simulink model "atlas_joint_impctrl_sqrt_damping_test"  (Simulink 8.5)
settings: Solver=ode4  StartTime=0.0  StopTime=2.0  FixedStep=1e-4  RelTol=1e-3
values from neighbouring files (symbols this model uses):
  B = d - 0.1*ones(NJL,1)    [atlas_joint_impctrl_sqrt_damping_test_settings_default.m]
  D = 0.7*eye(NJL)    [atlas_joint_impctrl_sqrt_damping_test_settings_default.m]
  F_ext_noise = 3    [atlas_joint_impctrl_sqrt_damping_test_settings_default.m]
  F_ext_noise_seed = 0    [atlas_joint_impctrl_sqrt_damping_test_settings_default.m]
  F_ext_noise_switch = 0    [atlas_joint_impctrl_sqrt_damping_test_settings_default.m]
  g_noise = 0.001    [atlas_joint_impctrl_sqrt_damping_test_settings_default.m]
  g_noise_seed = 0    [atlas_joint_impctrl_sqrt_damping_test_settings_default.m]
  g_noise_switch = 0    [atlas_joint_impctrl_sqrt_damping_test_settings_default.m]
  q_noise = 0.01    [atlas_joint_impctrl_sqrt_damping_test_settings_default.m]
  q_noise_seed = 0    [atlas_joint_impctrl_sqrt_damping_test_settings_default.m]
  q_noise_switch = 0    [atlas_joint_impctrl_sqrt_damping_test_settings_default.m]
  qD_noise = 0.01    [atlas_joint_impctrl_sqrt_damping_test_settings_default.m]
  qD_noise_seed = 0    [atlas_joint_impctrl_sqrt_damping_test_settings_default.m]
  qD_noise_switch = 0    [atlas_joint_impctrl_sqrt_damping_test_settings_default.m]
  T = 0.001    [atlas_joint_impctrl_sqrt_damping_test_settings_default.m]
  tau_noise = 0.5    [atlas_joint_impctrl_sqrt_damping_test_settings_default.m]
  tau_noise_seed = 0    [atlas_joint_impctrl_sqrt_damping_test_settings_default.m]
  tau_noise_switch = 0    [atlas_joint_impctrl_sqrt_damping_test_settings_default.m]
undefined symbols (not defined in the file): T1_filter_input, T1_filter_output
libraries: atlas_dynamic_library x5, atlas_impctrl_library x2
settings Model: Creator=knoechelmann  LastModifiedBy=Vorndamme  SimulationMode=rapid-accelerator  CovSFcnEnable=off
settings DataIOCC: LimitDataPoints=off  SaveFormat=StructureWithTime  SignalLoggingSaveFormat=Dataset
settings OptimizationCC: ExpressionDepthLimit=128
settings DebuggingCC: SignalInfNanChecking=warning  SignalRangeChecking=warning  UnderspecifiedInitializationDetection=Simplified  MergeDetectMultiDrivingBlocksExec=error  SolverPrmCheckMsg=warning  MultiTaskRateTransMsg=warning  CheckMatrixSingularityMsg=warning  UnderSpecifiedDataTypeMsg=warning  FcnCallInpInsideContextMsg=EnableAllAsError  StateNameClashWarn=none
settings GRTTargetCC: CombineOutputUpdateFcns=on  GRTInterface=off

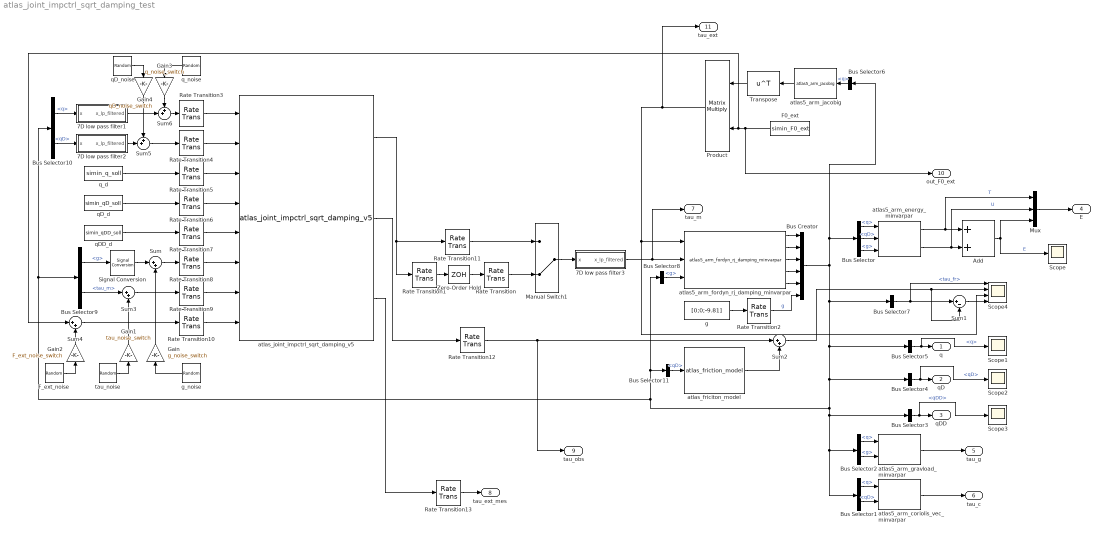
== system atlas_joint_impctrl_sqrt_damping_test ==
  7D low pass filter1 : Subsystem  mask{f=T1_filter_input}
      mask prompts: f "T1"
  7D low pass filter2 : Subsystem  mask{f=T1_filter_input}
      mask prompts: f "T1"
  7D low pass filter3 : Subsystem  mask{f=T1_filter_output}
      mask prompts: f "T1"
  Add : Sum
  Bus Creator : BusCreator  Inputs='q','qD','qDD','tau_fr','tau_m','g'
  Bus Selector : BusSelector  OutputSignals=q,qD,g
  Bus Selector1 : BusSelector  OutputSignals=q,qD
  Bus Selector10 : BusSelector  OutputSignals=q,qD
  Bus Selector11 : BusSelector  OutputSignals=qD
  Bus Selector2 : BusSelector  OutputSignals=q,g
  Bus Selector3 : BusSelector  OutputSignals=qDD
  Bus Selector4 : BusSelector  OutputSignals=qD
  Bus Selector5 : BusSelector  OutputSignals=q
  Bus Selector6 : BusSelector  OutputSignals=q
  Bus Selector7 : BusSelector  OutputSignals=tau_fr
  Bus Selector8 : BusSelector  OutputSignals=g
  Bus Selector9 : BusSelector  OutputSignals=g,tau_m
  F0_ext : FromWorkspace  VariableName=simin_F0_ext  SampleTime=0  Interpolate=off  OutputAfterFinalValue=Holding final value
  F_ext_noise : UniformRandomNumber  Minimum=-F_ext_noise  Maximum=F_ext_noise  Seed=F_ext_noise_seed  SampleTime=0
  Gain : Gain  Gain=g_noise_switch
  Gain1 : Gain  Gain=tau_noise_switch
  Gain2 : Gain  Gain=F_ext_noise_switch
  Gain3 : Gain  Gain=q_noise_switch
  Gain4 : Gain  Gain=qD_noise_switch
  Manual Switch1 : ManualSwitch  CurrentSetting=0
  Mux : Mux  Inputs=3
  Product : Product  Multiplication=Matrix(*)
  Rate Transition{,1..13} (14 alike) : RateTransition
  Scope{,1..3} (4 alike) : Scope
      Scope2 settings: SaveName=ScopeData2
      Scope3 settings: SaveName=ScopeData3
  Scope4 : Scope  NumInputPorts=4
      settings: YMin=-15~-1~-1~-40  YMax=15~1~1~40  SaveName=ScopeData4
  Signal Conversion : SignalConversion
  Sum{,2..4} (4 alike) : Sum  Inputs=|++
  Sum1 : Sum  Inputs=|+-
  Sum5 : Sum  Inputs=++|
  Sum6 : Sum  Inputs=++|
  Transpose : Math  Operator=transpose  SaturateOnIntegerOverflow=on
  Zero-Order Hold : ZeroOrderHold  SampleTime=0.001
  atlas5_arm_coriolis_vec_minvarpar : atlas_dynamic_library/atlas5_arm_coriolis_vec_minvarpar  atlas_arm_lr=atlas_arm_lr  MPV=MPV_arm_plant
  atlas5_arm_energy_minvarpar : atlas_dynamic_library/atlas5_arm_energy_minvarpar  MPV=MPV_arm_plant
  atlas5_arm_fordyn_rj_damping_minvarpar : atlas_dynamic_library/atlas5_arm_fordyn_rj_damping_minvarpar  q0=q0  qD0=qD0  d=d  muC=muC  atlas_arm_lr=atlas_arm_lr  MPV=MPV_arm_plant
  atlas5_arm_gravload_minvarpar : atlas_dynamic_library/atlas5_arm_gravload_minvarpar  atlas_arm_lr=atlas_arm_lr  MPV=MPV_arm_plant
  atlas5_arm_jacobig : atlas_dynamic_library/atlas5_arm_jacobig
  atlas_friciton_model : atlas_impctrl_library/atlas_friction_model  tau_c=tau_c  B=B
  atlas_joint_impctrl_sqrt_damping_v5 : atlas_impctrl_library/atlas_joint_impctrl_sqrt_damping_v5  K_d=K_d  D=D  K_tau_g=K_tau_g  K_tau_c=K_tau_c  K_tau_K=K_tau_K  K_tau_D=K_tau_D  K_tau_a=K_tau_a  K_tau_f=K_tau_f  K_tau_e=K_tau_e  K_tau_o=K_tau_o  K_qD_d=K_qD_d  K_qDD_d=K_qDD_d  K_ext_c=K_ext_c  K_obs_c=K_obs_c  K_fri_o=K_fri_o  K_ext_o=K_ext_o  MPV_arm_damp=MPV_arm_damp  MPV_arm_model=MPV_arm_model  tau_c=tau_c  B=B  qD_th=qD_th  tau_th=tau_th  K_O=K_O  T=T  atlas_arm_lr=atlas_arm_lr  T1=T1
  g : Constant  Value=[0;0;-9.81]
  g_noise : UniformRandomNumber  Minimum=-g_noise  Maximum=g_noise  Seed=g_noise_seed  SampleTime=0
  qDD_d : FromWorkspace  VariableName=simin_qDD_soll  SampleTime=0  OutputAfterFinalValue=Holding final value
  qD_d : FromWorkspace  VariableName=simin_qD_soll  SampleTime=0  OutputAfterFinalValue=Holding final value
  qD_noise : UniformRandomNumber  Minimum=-qD_noise  Maximum=qD_noise  Seed=qD_noise_seed  SampleTime=0
  q_d : FromWorkspace  VariableName=simin_q_soll  SampleTime=0  OutputAfterFinalValue=Holding final value
  q_noise : UniformRandomNumber  Minimum=-q_noise  Maximum=q_noise  Seed=q_noise_seed  SampleTime=0
  tau_noise : UniformRandomNumber  Minimum=-tau_noise  Maximum=tau_noise  Seed=tau_noise_seed  SampleTime=0
  q : Outport
  qD : Outport  Port=2
  qDD : Outport  Port=3
  E : Outport  Port=4
  tau_g : Outport  Port=5
  tau_c : Outport  Port=6
  tau_m : Outport  Port=7
  tau_ext_mes : Outport  Port=8
  tau_obs : Outport  Port=9
  out_F0_ext : Outport  Port=10
  tau_ext : Outport  Port=11
  wires:
  atlas5_arm_energy_minvarpar/1 -> Mux/1, Add/1  "T"
  atlas5_arm_energy_minvarpar/2 -> Mux/2, Add/2  "U"
  Add/1 -> Scope/1, Mux/3  "E"
  atlas5_arm_jacobig/1 -> Transpose/1
  Product/1 -> tau_ext/1, atlas5_arm_fordyn_rj_damping_minvarpar/1, Scope4/3
  F0_ext/1 -> out_F0_ext/1, Sum4/1, Product/2
  atlas5_arm_gravload_minvarpar/1 -> tau_g/1
  atlas5_arm_coriolis_vec_minvarpar/1 -> tau_c/1
  qD_d/1 -> Rate Transition6/1
  qDD_d/1 -> Rate Transition7/1
  q_d/1 -> Rate Transition5/1
  Manual Switch1/1 -> 7D low pass filter3/1(x)
  atlas_joint_impctrl_sqrt_damping_v5/1 -> Rate Transition1/1, Rate Transition11/1
  Rate Transition1/1 -> Zero-Order Hold/1
  Zero-Order Hold/1 -> Rate Transition/1
  Rate Transition/1 -> Manual Switch1/2
  7D low pass filter3/1(x_lp_filtered) -> tau_m/1, atlas5_arm_fordyn_rj_damping_minvarpar/2
  atlas_joint_impctrl_sqrt_damping_v5/2 -> Rate Transition12/1
  Sum1/1 -> Scope4/4
  Transpose/1 -> Product/1
  atlas5_arm_fordyn_rj_damping_minvarpar/1 -> Bus Creator/1
  atlas5_arm_fordyn_rj_damping_minvarpar/2 -> Bus Creator/2
  atlas5_arm_fordyn_rj_damping_minvarpar/3 -> Bus Creator/3
  Bus Selector/2 -> atlas5_arm_energy_minvarpar/2  "<qD>"
  Bus Selector/1 -> atlas5_arm_energy_minvarpar/1  "<q>"
  Bus Creator/1 -> Bus Selector5/1, Bus Selector8/1, Bus Selector11/1, Bus Selector10/1, Bus Selector9/1, Bus Selector1/1, Bus Selector2/1, Bus Selector3/1, Bus Selector4/1, Bus Selector7/1, Bus Selector6/1, Bus Selector/1
  Bus Selector1/1 -> atlas5_arm_coriolis_vec_minvarpar/1  "<q>"
  Bus Selector1/2 -> atlas5_arm_coriolis_vec_minvarpar/2  "<qD>"
  Bus Selector2/1 -> atlas5_arm_gravload_minvarpar/1  "<q>"
  atlas5_arm_fordyn_rj_damping_minvarpar/4 -> Bus Creator/4
  g/1 -> Rate Transition2/1
  Rate Transition2/1 -> Bus Creator/6  "g"
  Bus Selector6/1 -> atlas5_arm_jacobig/1  "<q>"
  Bus Selector7/1 -> Scope4/1, Sum1/1  "<tau_fr>"
  Bus Selector5/1 -> Scope1/1, q/1  "<q>"
  Bus Selector4/1 -> Scope2/1, qD/1  "<qD>"
  Bus Selector3/1 -> Scope3/1, qDD/1  "<qDD>"
  Bus Selector2/2 -> atlas5_arm_gravload_minvarpar/2  "<g>"
  Bus Selector/3 -> atlas5_arm_energy_minvarpar/3  "<g>"
  Bus Selector8/1 -> atlas5_arm_fordyn_rj_damping_minvarpar/3  "<g>"
  Bus Selector9/1 -> Signal Conversion/1  "<g>"
  Bus Selector10/1 -> 7D low pass filter1/1(x)  "<q>"
  Bus Selector10/2 -> 7D low pass filter2/1(x)  "<qD>"
  atlas5_arm_fordyn_rj_damping_minvarpar/5 -> Bus Creator/5
  Rate Transition3/1 -> atlas_joint_impctrl_sqrt_damping_v5/1
  Rate Transition4/1 -> atlas_joint_impctrl_sqrt_damping_v5/2
  Rate Transition5/1 -> atlas_joint_impctrl_sqrt_damping_v5/3
  Rate Transition6/1 -> atlas_joint_impctrl_sqrt_damping_v5/4
  Rate Transition7/1 -> atlas_joint_impctrl_sqrt_damping_v5/5
  Rate Transition8/1 -> atlas_joint_impctrl_sqrt_damping_v5/6
  Rate Transition9/1 -> atlas_joint_impctrl_sqrt_damping_v5/7
  Rate Transition10/1 -> atlas_joint_impctrl_sqrt_damping_v5/8
  Rate Transition11/1 -> Manual Switch1/1
  Rate Transition12/1 -> tau_obs/1, Sum2/1
  Bus Selector11/1 -> atlas_friciton_model/1  "<qD>"
  atlas_friciton_model/1 -> Sum2/2
  Sum2/1 -> Sum1/2, Scope4/2
  atlas_joint_impctrl_sqrt_damping_v5/3 -> Rate Transition13/1
  Mux/1 -> E/1
  Rate Transition13/1 -> tau_ext_mes/1
  Signal Conversion/1 -> Sum/1
  Sum/1 -> Rate Transition8/1
  g_noise/1 -> Gain/1
  Bus Selector9/2 -> Sum3/1  "<tau_m>"
  Sum3/1 -> Rate Transition9/1
  tau_noise/1 -> Gain1/1
  Sum4/1 -> Rate Transition10/1
  F_ext_noise/1 -> Gain2/1
  7D low pass filter2/1(x_lp_filtered) -> Sum5/2
  Sum5/1 -> Rate Transition4/1
  7D low pass filter1/1(x_lp_filtered) -> Sum6/2
  Sum6/1 -> Rate Transition3/1
  q_noise/1 -> Gain3/1
  qD_noise/1 -> Gain4/1
  Gain/1 -> Sum/2
  Gain1/1 -> Sum3/2
  Gain2/1 -> Sum4/2
  Gain3/1 -> Sum6/1
  Gain4/1 -> Sum5/1

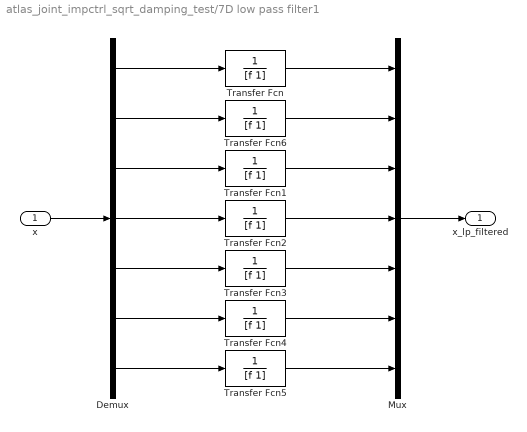
== system atlas_joint_impctrl_sqrt_damping_test/7D low pass filter1 ==
  x : Inport
  Demux : Demux  Outputs=7
  Mux : Mux  Inputs=7
  Transfer Fcn{,1..6} (7 alike) : TransferFcn  Denominator=[f 1]
  x_lp_filtered : Outport
  wires:
  x/1 -> Demux/1
  Mux/1 -> x_lp_filtered/1
  Demux/1 -> Transfer Fcn/1
  Transfer Fcn/1 -> Mux/1
  Demux/6 -> Transfer Fcn4/1
  Transfer Fcn4/1 -> Mux/6
  Demux/2 -> Transfer Fcn6/1
  Transfer Fcn6/1 -> Mux/2
  Demux/3 -> Transfer Fcn1/1
  Transfer Fcn1/1 -> Mux/3
  Demux/4 -> Transfer Fcn2/1
  Transfer Fcn2/1 -> Mux/4
  Demux/5 -> Transfer Fcn3/1
  Transfer Fcn3/1 -> Mux/5
  Demux/7 -> Transfer Fcn5/1
  Transfer Fcn5/1 -> Mux/7

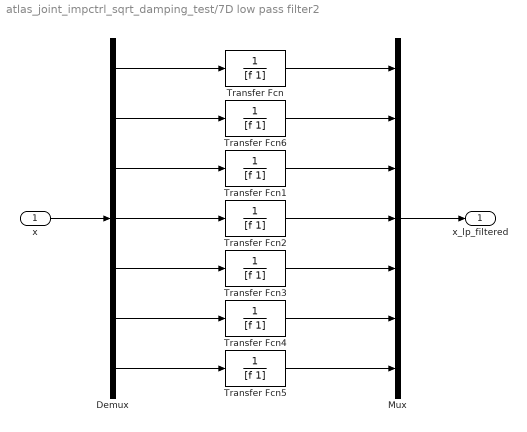
== system atlas_joint_impctrl_sqrt_damping_test/7D low pass filter2 ==
  x : Inport
  Demux : Demux  Outputs=7
  Mux : Mux  Inputs=7
  Transfer Fcn{,1..6} (7 alike) : TransferFcn  Denominator=[f 1]
  x_lp_filtered : Outport
  wires:
  x/1 -> Demux/1
  Mux/1 -> x_lp_filtered/1
  Demux/1 -> Transfer Fcn/1
  Transfer Fcn/1 -> Mux/1
  Demux/6 -> Transfer Fcn4/1
  Transfer Fcn4/1 -> Mux/6
  Demux/2 -> Transfer Fcn6/1
  Transfer Fcn6/1 -> Mux/2
  Demux/3 -> Transfer Fcn1/1
  Transfer Fcn1/1 -> Mux/3
  Demux/4 -> Transfer Fcn2/1
  Transfer Fcn2/1 -> Mux/4
  Demux/5 -> Transfer Fcn3/1
  Transfer Fcn3/1 -> Mux/5
  Demux/7 -> Transfer Fcn5/1
  Transfer Fcn5/1 -> Mux/7

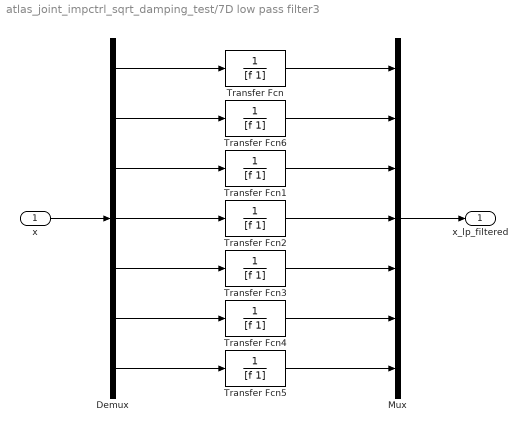
== system atlas_joint_impctrl_sqrt_damping_test/7D low pass filter3 ==
  x : Inport
  Demux : Demux  Outputs=7
  Mux : Mux  Inputs=7
  Transfer Fcn{,1..6} (7 alike) : TransferFcn  Denominator=[f 1]
  x_lp_filtered : Outport
  wires:
  x/1 -> Demux/1
  Mux/1 -> x_lp_filtered/1
  Demux/1 -> Transfer Fcn/1
  Transfer Fcn/1 -> Mux/1
  Demux/6 -> Transfer Fcn4/1
  Transfer Fcn4/1 -> Mux/6
  Demux/2 -> Transfer Fcn6/1
  Transfer Fcn6/1 -> Mux/2
  Demux/3 -> Transfer Fcn1/1
  Transfer Fcn1/1 -> Mux/3
  Demux/4 -> Transfer Fcn2/1
  Transfer Fcn2/1 -> Mux/4
  Demux/5 -> Transfer Fcn3/1
  Transfer Fcn3/1 -> Mux/5
  Demux/7 -> Transfer Fcn5/1
  Transfer Fcn5/1 -> Mux/7
